simulink model "MMA"  (R2020a)
settings: Solver=VariableStepAuto  StartTime=0.0  StopTime=10.0  RelTol=1e-3
values from neighbouring files (symbols this model uses):
  b = 1.5    [Sistema_MMA.m]
  g = 9.81    [Sistema_MMA.m]
  k = 20    [Sistema_MMA.m]
  m = 3    [Sistema_MMA.m]
settings Model: Creator=gabri  LastModifiedBy=gabri

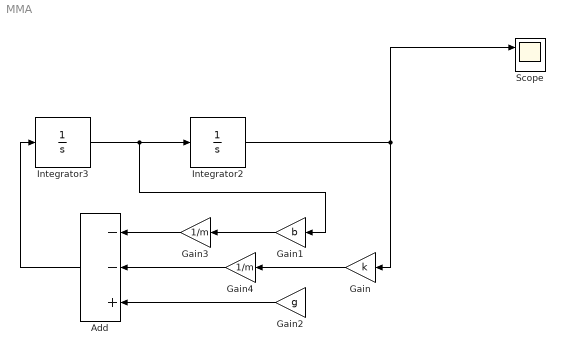
== system MMA ==
  Add : Sum  Inputs=--+
  Gain : Gain  Gain=k
  Gain1 : Gain  Gain=b
  Gain2 : Gain  Gain=g
  Gain3 : Gain  Gain=1/m
  Gain4 : Gain  Gain=1/m
  Integrator2 : Integrator  InitialCondition=10
  Integrator3 : Integrator
  Scope : Scope  NumInputPorts=2
  wires:
  Integrator2/1 -> Gain/1, Scope/1
  Add/1 -> Integrator3/1
  Integrator3/1 -> Gain1/1, Integrator2/1
  Gain2/1 -> Add/3
  Gain1/1 -> Gain3/1
  Gain3/1 -> Add/1
  Gain/1 -> Gain4/1
  Gain4/1 -> Add/2
